simulink model "test_01_cacc_sim"  (R2022b)
settings: Solver=VariableStepAuto  StartTime=0.0  StopTime=100  RelTol=1e-3
values from neighbouring files (symbols this model uses):
  accel = [1 0 1 0 -1 0 -0.5 0]    [cacc_test_01.m]    (also in test_01_cacc.m = [1 0 -1 0 -1 0 1 0]; test_02_cacc.m = [1 0 -1 0 -1 0 1 0]; test_04_cacc_hete.m = [traction_accel 0 bracking_accel 0 bracking_accel 0 traction; test_04_cacc_homo.m = [traction_accel 0 bracking_accel 0 bracking_accel 0 traction)
  e_init = [2 -1 -2]    [cacc_test_01.m]    (also in test_01_cacc.m; test_02_cacc.m; test_04_cacc_hete.m = [e_init1 e_init2 e_init3]; test_04_cacc_homo.m = [e_init1 e_init2 e_init3])
  m1 = 1460    [cacc_test_01.m]    (also in test_01_cacc.m; test_02_cacc.m)
  m2 = 1460    [cacc_test_01.m]    (also in test_01_cacc.m; test_02_cacc.m)
  m3 = 1460    [cacc_test_01.m]    (also in test_01_cacc.m; test_02_cacc.m)
  sim_mode = 1    [test_01_cacc.m]    (also in test_02_cacc.m; test_04_cacc_hete.m; test_04_cacc_homo.m; test_05_cacc_hete.m)
  v_ref0 = 0    [cacc_test_01.m]    (also in test_01_cacc.m; test_02_cacc.m; test_04_cacc_hete.m = 5; test_04_cacc_homo.m = 5)
  wp = tril(ones(length(dt)))*dt    [cacc_test_01.m]    (also in test_01_cacc.m; test_02_cacc.m; test_04_cacc_hete.m; test_04_cacc_homo.m)
libraries: cstblocks x6
settings Model: Creator=phatdo  LastModifiedBy=phatdo
settings DataIOCC: ReturnWorkspaceOutputs=off

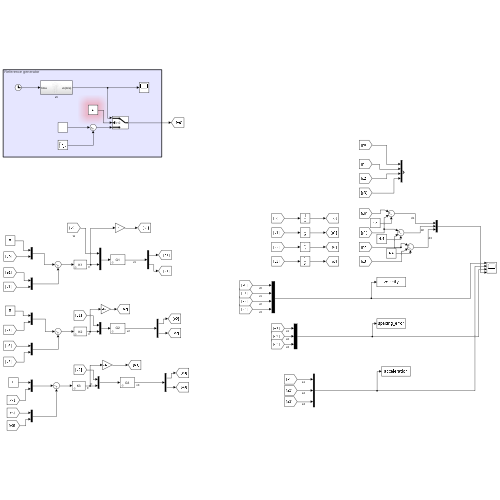
[thumbnail: Simulink's stored preview of the top-level diagram]
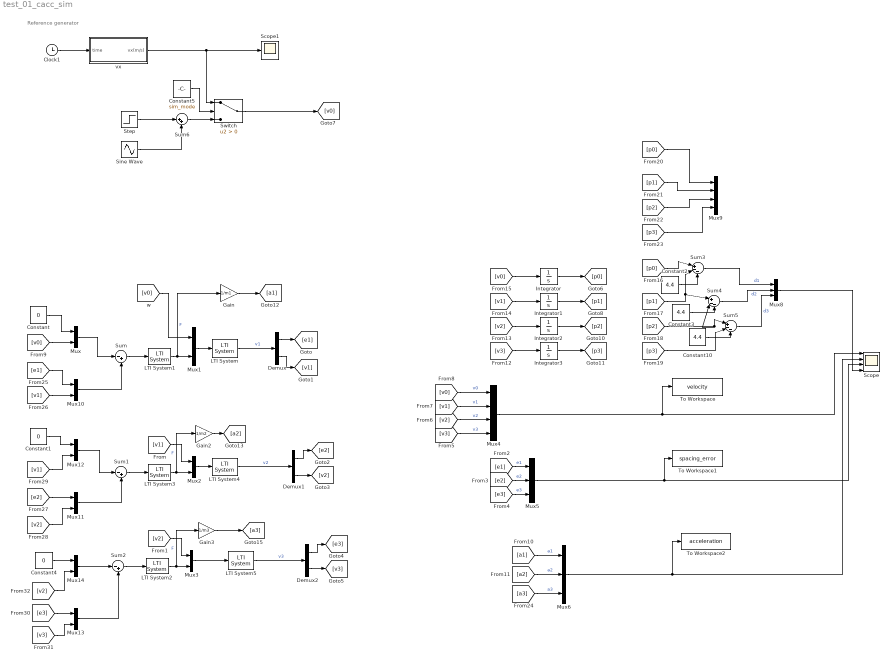
== system test_01_cacc_sim ==
  note: Reference generator
  Clock1 : Clock
  Constant : Constant  Value=0
  Constant1 : Constant  Value=0
  Constant10 : Constant  Value=4.4
  Constant2 : Constant  Value=4.4
  Constant3 : Constant  Value=4.4
  Constant4 : Constant  Value=0
  Constant5 : Constant  Value=sim_mode
  Demux : Demux  Outputs=2
  Demux1 : Demux  Outputs=2
  Demux2 : Demux  Outputs=2
  Gain : Gain  Gain=1/m1
  Gain2 : Gain  Gain=1/m2
  Gain3 : Gain  Gain=1/m3
  Integrator : Integrator
  Integrator1 : Integrator  InitialCondition=-e_init(1)
  Integrator2 : Integrator  InitialCondition=-e_init(2)-e_init(1)
  Integrator3 : Integrator  InitialCondition=-e_init(2)-e_init(1)-e_init(3)
  LTI System : cstblocks/LTI System  sys=G1  IC=[e_init(1) 0]
  LTI System1 : cstblocks/LTI System  sys=K1  IC=[]
  LTI System2 : cstblocks/LTI System  sys=K3  IC=[]
  LTI System3 : cstblocks/LTI System  sys=K2  IC=[]
  LTI System4 : cstblocks/LTI System  sys=G2  IC=[e_init(2) 0]
  LTI System5 : cstblocks/LTI System  sys=G3  IC=[e_init(3) 0]
  Mux{,1..3,10..14} (9 alike) : Mux  Inputs=2
  Mux4 : Mux
  Mux5 : Mux  Inputs=3
  Mux6 : Mux  Inputs=3
  Mux8 : Mux  Inputs=3
  Mux9 : Mux
  Scope : Scope  NumInputPorts=4
  Scope1 : Scope
  Sine Wave : Sin  Amplitude=5  Frequency=0.5  SampleTime=0
  Step : Step  Time=0  After=15  SampleTime=0
  Sum : Sum  Inputs=|-+
  Sum1 : Sum  Inputs=|-+
  Sum2 : Sum  Inputs=|-+
  Sum3 : Sum  Inputs=|+--
  Sum4 : Sum  Inputs=|+--
  Sum5 : Sum  Inputs=|+--
  Sum6 : Sum  Inputs=|++
  Switch : Switch  Criteria=u2 > Threshold  SaturateOnIntegerOverflow=off  InputSameDT=off
  To Workspace : ToWorkspace  VariableName=velocity  SaveFormat=Timeseries  SampleTime=-1
  To Workspace1 : ToWorkspace  VariableName=spacing_error  SaveFormat=Timeseries  SampleTime=-1
  To Workspace2 : ToWorkspace  VariableName=acceleration  SaveFormat=Timeseries  SampleTime=-1
  vx : Subsystem
  wires:
  Sum/1 -> LTI System1/1
  Sum1/1 -> LTI System3/1
  Sum2/1 -> LTI System2/1
  LTI System4/1 -> Demux1/1  "v2"
  LTI System5/1 -> Demux2/1  "v3"
  Mux1/1 -> LTI System/1
  LTI System1/1 -> Mux1/2, Gain/1  "F"
  Mux2/1 -> LTI System4/1
  Mux3/1 -> LTI System5/1
  LTI System3/1 -> Mux2/2, Gain2/1  "F"
  LTI System/1 -> Demux/1  "v1"
  Constant/1 -> Mux/1
  Mux4/1 -> To Workspace/1, Scope/1
  Demux/1 -> [e1]
  Demux/2 -> [v1]
  [v1] -> Mux2/1
  Demux1/1 -> [e2]
  Demux1/2 -> [v2]
  Demux2/1 -> [e3]
  Demux2/2 -> [v3]
  [v2] -> Mux3/1
  [v0] -> Mux4/1  "v0"
  [v1] -> Mux4/2  "v1"
  [v2] -> Mux4/3  "v2"
  [v3] -> Mux4/4  "v3"
  Mux5/1 -> Scope/3, To Workspace1/1
  [e1] -> Mux5/1  "e1"
  [e2] -> Mux5/2  "e2"
  [e3] -> Mux5/3  "e3"
  [v0] -> Mux1/1
  [v0] -> Mux/2
  [v0] -> Integrator/1
  [v1] -> Integrator1/1
  [v2] -> Integrator2/1
  [v3] -> Integrator3/1
  Integrator/1 -> [p0]
  Integrator1/1 -> [p1]
  Integrator2/1 -> [p2]
  Integrator3/1 -> [p3]
  [p0] -> Sum3/1
  [p1] -> Sum4/1, Sum3/2
  [p2] -> Sum5/1, Sum4/2
  [p3] -> Sum5/2
  Sum3/1 -> Mux8/1  "d1"
  Sum4/1 -> Mux8/2  "d2"
  Sum5/1 -> Mux8/3  "d3"
  Mux8/1 -> Scope/4
  [p0] -> Mux9/1
  [p1] -> Mux9/2
  [p2] -> Mux9/3
  [p3] -> Mux9/4
  Constant2/1 -> Sum3/3
  Constant3/1 -> Sum4/3
  Constant10/1 -> Sum5/3
  Gain/1 -> [a1]
  Gain2/1 -> [a2]
  Gain3/1 -> [a3]
  LTI System2/1 -> Gain3/1, Mux3/2  "F"
  [a1] -> Mux6/1  "a1"
  [a2] -> Mux6/2  "a2"
  [a3] -> Mux6/3  "a3"
  Mux6/1 -> To Workspace2/1, Scope/2
  Clock1/1 -> vx/1(time)
  vx/1(vx(m/s)) -> Scope1/1, Switch/1
  [e1] -> Mux10/1
  [v1] -> Mux10/2
  Mux10/1 -> Sum/2
  Mux/1 -> Sum/1
  Constant1/1 -> Mux12/1
  Mux12/1 -> Sum1/1
  [v1] -> Mux12/2
  [e2] -> Mux11/1
  [v2] -> Mux11/2
  Mux11/1 -> Sum1/2
  [e3] -> Mux13/1
  [v3] -> Mux13/2
  Mux13/1 -> Sum2/2
  Constant4/1 -> Mux14/1
  Mux14/1 -> Sum2/1
  [v2] -> Mux14/2
  Step/1 -> Sum6/1
  Sine Wave/1 -> Sum6/2
  Constant5/1 -> Switch/2
  Switch/1 -> [v0]
  Sum6/1 -> Switch/3

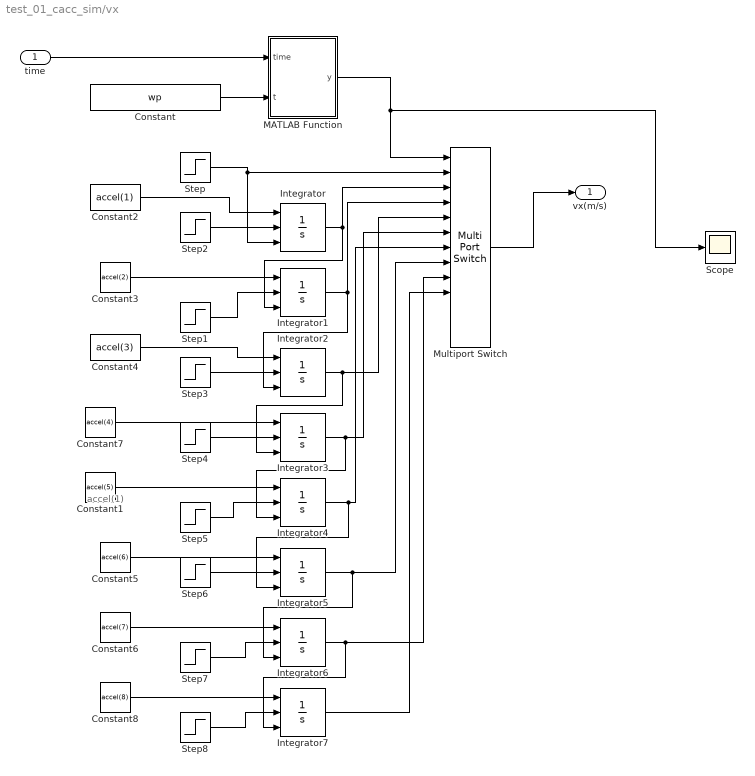
== system test_01_cacc_sim/vx ==
  note: accel(1)
  time : Inport  SampleTime=0.08
  Constant : Constant  Value=wp
  Constant1 : Constant  Value=accel(5)
  Constant2 : Constant  Value=accel(1)
  Constant3 : Constant  Value=accel(2)
  Constant4 : Constant  Value=accel(3)
  Constant5 : Constant  Value=accel(6)
  Constant6 : Constant  Value=accel(7)
  Constant7 : Constant  Value=accel(4)
  Constant8 : Constant  Value=accel(8)
  Integrator{,1..7} (8 alike) : Integrator  ExternalReset=rising  InitialConditionSource=external
  MATLAB Function : MATLAB Function  TreatAsAtomicUnit=on
  Multiport Switch : MultiPortSwitch  Inputs=12  SaturateOnIntegerOverflow=off  InputSameDT=off
  Scope : Scope
  Step : Step  Time=0  Before=v_ref0  After=v_ref0  SampleTime=0
  Step1 : Step  Time=wp(2)  SampleTime=0
  Step2 : Step  Time=wp(1)  SampleTime=0
  Step3 : Step  Time=wp(3)  SampleTime=0
  Step4 : Step  Time=wp(4)  SampleTime=0
  Step5 : Step  Time=wp(5)  SampleTime=0
  Step6 : Step  Time=wp(6)  SampleTime=0
  Step7 : Step  Time=wp(7)  SampleTime=0
  Step8 : Step  Time=wp(8)  SampleTime=0
  vx(m/s) : Outport
  wires:
  Step/1 -> Integrator/3, Multiport Switch/2
  Constant/1 -> MATLAB Function/2(t)
  Constant2/1 -> Integrator/1
  Multiport Switch/1 -> vx(m/s)/1
  Integrator/1 -> Integrator1/3, Multiport Switch/3
  Step2/1 -> Integrator/2
  Constant3/1 -> Integrator1/1
  Integrator1/1 -> Integrator2/3, Multiport Switch/4
  Step1/1 -> Integrator1/2
  time/1 -> MATLAB Function/1(time)
  Step3/1 -> Integrator2/2
  Constant4/1 -> Integrator2/1
  Integrator2/1 -> Integrator3/3, Multiport Switch/5
  Integrator3/1 -> Integrator4/3, Multiport Switch/6
  Step4/1 -> Integrator3/2
  Constant7/1 -> Integrator3/1
  MATLAB Function/1(y) -> Scope/1, Multiport Switch/1
  Integrator4/1 -> Integrator5/3, Multiport Switch/7
  Step5/1 -> Integrator4/2
  Step6/1 -> Integrator5/2
  Constant1/1 -> Integrator4/1
  Constant5/1 -> Integrator5/1
  Integrator5/1 -> Integrator6/3, Multiport Switch/8
  Step7/1 -> Integrator6/2
  Constant6/1 -> Integrator6/1
  Constant8/1 -> Integrator7/1
  Step8/1 -> Integrator7/2
  Integrator6/1 -> Integrator7/3, Multiport Switch/9
  Integrator7/1 -> Multiport Switch/10

== matlab function test_01_cacc_sim/vx/MATLAB Function ==
  data: time input; t input; y output
function y = fcn(time,t)
t1 = t(1);
t2 = t(2);
t3 = t(3);
t4 = t(4);
t5 = t(5);
t6 = t(6);
t7 = t(7);
t8 = t(8);

if time<=t1
    y = 1;
elseif time>t1 && time <= t2
    y = 2;
elseif time>t2 && time <= t3
    y = 3;
elseif time>t3 && time <= t4
    y = 4;
elseif time>t4 && time <= t5
    y = 5;
elseif time>t5 && time <= t6
    y = 6;
elseif time>t6 && time <= t7
    y = 7;
elseif time>t7 && time <= t8
    y = 8;
else 
    y = 9;
end
